simulink model "PI_Controller"  (R2018a)
settings: Solver=VariableStepAuto  StartTime=0.0  StopTime=35  RelTol=1e-3
undefined symbols (not defined in the file): D1, lagging, pulse
libraries: powerlib x12, powerlib_meascontrol x2, simulink x1
settings Model: Creator=Gulten  LastModifiedBy=Gulten

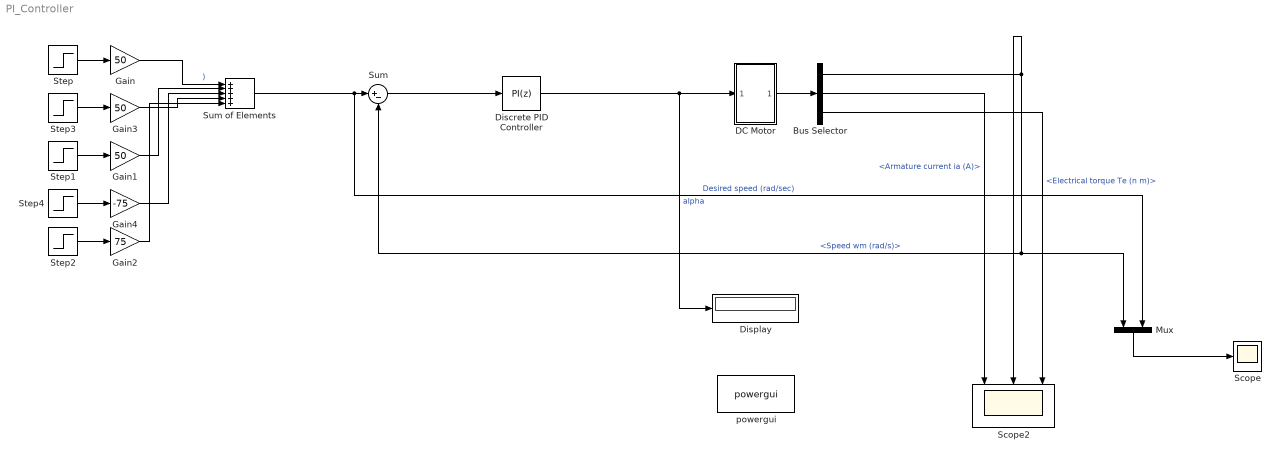
== system PI_Controller ==
  Bus Selector : BusSelector  OutputSignals=Speed wm (rad/s),Armature current ia (A),Electrical torque Te (n m)
  DC Motor : Subsystem
  Discrete PID Controller : simulink/Continuous/PID Controller  Controller=PI  TimeDomain=Discrete-time  SampleTime=0.001  IntegratorMethod=Forward Euler  FilterMethod=Forward Euler  Form=Parallel  UseFilter=on  ControllerParametersSource=internal  P=-2.0474  I=-3.7917  D=0  N=100  InitialConditionSource=internal  InitialConditionForIntegrator=0  InitialConditionForFilter=0  ExternalReset=none  IgnoreLimit=on  LimitOutput=on  UpperSaturationLimit=90  LowerSaturationLimit=0  LinearizeAsGain=off  AntiWindupMode=none  Kb=1  TrackingMode=off  Kt=1  PParamMin=[]  PParamMax=[]  IParamMin=[]  IParamMax=[]  DParamMin=[]  DParamMax=[]  NParamMin=[]  NParamMax=[]  KbParamMin=[]  KbParamMax=[]  KtParamMin=[]  KtParamMax=[]  POutMin=[]  POutMax=[]  IOutMin=[]  IOutMax=[]  DOutMin=[]  DOutMax=[]  NOutMin=[]  NOutMax=[]  KbOutMin=[]  KbOutMax=[]  KtOutMin=[]  KtOutMax=[]  IntegratorOutMin=[]  IntegratorOutMax=[]  FilterOutMin=[]  FilterOutMax=[]  SumOutMin=[]  SumOutMax=[]  SumI1OutMin=[]  SumI1OutMax=[]  SumI2OutMin=[]  SumI2OutMax=[]  SumI3OutMin=[]  SumI3OutMax=[]  SumDOutMin=[]  SumDOutMax=[]  SaturationOutMin=[]  SaturationOutMax=[]  IntegratorContinuousStateAttributes=''  IntegratorStateMustResolveToSignalObject=off  IntegratorRTWStateStorageClass=Auto  FilterContinuousStateAttributes=''  FilterStateMustResolveToSignalObject=off  FilterRTWStateStorageClass=Auto  DifferentiatorICPrevScaledInput=0  DifferentiatorOutMin=[]  DifferentiatorOutMax=[]  FilterDiffOutCoefMin=[]  FilterDiffOutCoefMax=[]  SumDenOutMin=[]  SumDenOutMax=[]  SumNumOutMin=[]  SumNumOutMax=[]  ReciprocalOutMin=[]  ReciprocalOutMax=[]  DivideOutMin=[]  DivideOutMax=[]  TunerSelectOption=Frequency Response Based
  Display : Display
  Gain : Gain  Gain=50
  Gain1 : Gain  Gain=50
  Gain2 : Gain  Gain=75
  Gain3 : Gain  Gain=50
  Gain4 : Gain  Gain=-75
  Mux : Mux  Inputs=2
  Scope : Scope
  Scope2 : Scope  NumInputPorts=3
  Step : Step  Time=0  SampleTime=0
  Step1 : Step  Time=5  SampleTime=0
  Step2 : Step  Time=25  SampleTime=0
  Step3 : Step  Time=3  SampleTime=0
  Step4 : Step  Time=15  SampleTime=0
  Sum : Sum  Inputs=|+-
  Sum of Elements : Sum  Inputs=+++++
  powergui : powerlib/powergui  Priority=1  SimulationMode=Discrete  SampleTime=10e-6  frequency=60  Iterations=50  frequencyindice=50  Pbase=100e6  ErrMax=1e-4  UnitsV=kV  UnitsW=MW  buscounter=0  FunctionMessages=off  echomessages=off  EnableUseOfTLC=off  CurrentSourceSwitches=off  DisableSnubberDevices=off  DisableRonSwitches=off  DisableVfSwitches=off  DisplayEquations=off  SolverType=Tustin/Backward Euler (TBE)  Interpol=off  ExternalGateDelay=off  methode=off  Ts=100  x0status=blocks  SPID=on  SwTol=0  HookPort=off  RestoreLinks=warning  ResistiveCurrentMeasurement=off  Frange=[0:2:500]  Ylog=off  Xlog=on  ShowGrid=off  save=off  variable=ZData  structure=ScopeData  ZoomFFT=on  StartTime=3  cycles=10  DisplayStyle=1  fundamental=50  FreqAxis=on  MaxFrequency=1000  frequencyindicesteady=1  RmsSteady=1  display=off
  wires:
  Bus Selector/3 -> Scope2/3  "<Electrical torque Te (n m)>"
  Bus Selector/1 -> Scope2/2, Mux/1, Sum/2  "<Speed wm (rad/s)>"
  Bus Selector/2 -> Scope2/1  "<Armature current ia (A)>"
  DC Motor/1(Out1) -> Bus Selector/1
  Step/1 -> Gain/1
  Mux/1 -> Scope/1
  Step1/1 -> Gain1/1
  Step2/1 -> Gain2/1
  Gain/1 -> Sum of Elements/1  ")"
  Gain1/1 -> Sum of Elements/2
  Gain2/1 -> Sum of Elements/5
  Sum of Elements/1 -> Mux/2, Sum/1  "Desired speed (rad/sec)"
  Discrete PID Controller/1 -> Display/1, DC Motor/1(In1)  "alpha"
  Sum/1 -> Discrete PID Controller/1
  Step3/1 -> Gain3/1
  Gain3/1 -> Sum of Elements/4
  Step4/1 -> Gain4/1
  Gain4/1 -> Sum of Elements/3

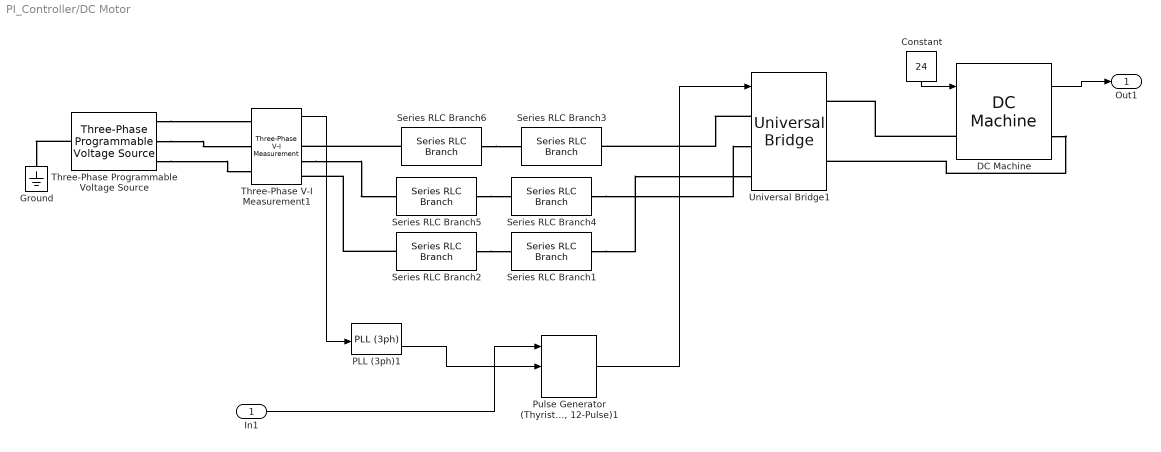
== system PI_Controller/DC Motor ==
  In1 : Inport
  Constant : Constant  Value=24
  DC Machine : powerlib/Machines/DC Machine  PresetModel=No  MechanicalLoad=Torque TL  FieldType=Permanent magnet  ShowDetailedParameters=on  MeasurementBus=off  RLa=[ 10 0.01]  RLf="[ 240  120]"  Laf=1.8  MachineConstant=Back-emf constant (V/rpm)  Ke=0.3  Kt=1.8  J=0.4  Bm=0  Tf=0  w0=1  Ifinit=1  TsPowergui=0  TsBlock=-1
  Ground : powerlib/Elements/Ground  LConnTagsString=a
  PLL (3ph)1 : powerlib_meascontrol/PLL/PLL (3ph)  Fmin=45  Par_Init=[0, 60]  ParK=[180, 3200, 1]  TcD=1e-4  MaxRateChangeFreq=12  FilterCutOffFreq=25  Ts=0  AGC=on
  "Pulse Generator (Thyristor, 12-Pulse)1" : powerlib_meascontrol/Pulse & Signal Generators/Pulse Generator (Thyristor, 12-Pulse)  GenType=6-pulse  Delta=D1 (lagging)  pwidth=60  Double_Pulse=off  Ts=1e-5
      settings: SourceProductName=Simscape Power Systems  SourceProductBaseCode=PS
  Series RLC Branch1 : powerlib/Elements/Series RLC Branch  LConnTagsString=__new0  RConnTagsString=__new0  BranchType=L  Resistance=1  Inductance=100e-6  SetiL0=off  InitialCurrent=0  Capacitance=1e-6  Setx0=off  InitialVoltage=0  Measurements=None
  Series RLC Branch2 : powerlib/Elements/Series RLC Branch  LConnTagsString=__new0  RConnTagsString=__new0  BranchType=R  Resistance=0.1  Inductance=1e-3  SetiL0=off  InitialCurrent=0  Capacitance=1e-6  Setx0=off  InitialVoltage=0  Measurements=None
  Series RLC Branch3 : powerlib/Elements/Series RLC Branch  LConnTagsString=__new0  RConnTagsString=__new0  BranchType=L  Resistance=1  Inductance=100e-6  SetiL0=off  InitialCurrent=0  Capacitance=1e-6  Setx0=off  InitialVoltage=0  Measurements=None
  Series RLC Branch4 : powerlib/Elements/Series RLC Branch  LConnTagsString=__new0  RConnTagsString=__new0  BranchType=L  Resistance=1  Inductance=100e-6  SetiL0=off  InitialCurrent=0  Capacitance=1e-6  Setx0=off  InitialVoltage=0  Measurements=None
  Series RLC Branch5 : powerlib/Elements/Series RLC Branch  LConnTagsString=__new0  RConnTagsString=__new0  BranchType=R  Resistance=0.1  Inductance=1e-3  SetiL0=off  InitialCurrent=0  Capacitance=1e-6  Setx0=off  InitialVoltage=0  Measurements=None
  Series RLC Branch6 : powerlib/Elements/Series RLC Branch  LConnTagsString=__new0  RConnTagsString=__new0  BranchType=R  Resistance=0.1  Inductance=1e-3  SetiL0=off  InitialCurrent=0  Capacitance=1e-6  Setx0=off  InitialVoltage=0  Measurements=None
  Three-Phase Programmable Voltage Source : powerlib/Electrical Sources/Three-Phase Programmable Voltage Source  PositiveSequence="[400  0 50]"  VariationEntity=None  VariationType=Table of time-amplitude pairs  VariationTypeAlt=Step  VariationStep=0.5  VariationRate=10  VariationMagnitude=0.3  VariationFrequency=2  VariationTiming=[1 2]  VariationPhaseA=off  Amplitudes=[1 0.8 1.2 1.0]  TimeValues=[0 0.1 0.15 0.2]  HarmonicGeneration=off  HarmonicA=[3 0.2 -25 0]  HarmonicB=[2 0.15 35 2]  Timing="[0.05  3]"  BusType=swing  Pref=0  Qref=0  Qmin=-inf  Qmax=inf
  Three-Phase V-I Measurement1 : powerlib/Measurements/Three-Phase V-I Measurement  VoltageMeasurement=phase-to-ground  SetLabelV=off  LabelV=Vabc  Vpu=off  VpuLL=off  CurrentMeasurement=yes  SetLabelI=off  LabelI=Iabc  Ipu=off  Pbase=100e6  Vbase=500e3  OutputType=Complex  PhasorSimulation=off  PSBequivalent=0
  Universal Bridge1 : powerlib/Power Electronics/Universal Bridge  Arms=3  SnubberResistance=1e5  SnubberCapacitance=inf  Device=Thyristors  Ron=0.020  Lon=0  ForwardVoltages="[  0  0  ]"  ForwardVoltage=0.8  GTOparameters=[ 10e-6 , 20e-6 ]  IGBTparameters=[ 1e-6 , 2e-6 ]  Measurements=None  Measurements_2=None  converterType=Rectifier
  Out1 : Outport
  wires:
  Constant/1 -> DC Machine/1
  "Pulse Generator (Thyristor, 12-Pulse)1"/1 -> Universal Bridge1/1
  PLL (3ph)1/2 -> "Pulse Generator (Thyristor, 12-Pulse)1"/2
  Three-Phase V-I Measurement1/1 -> PLL (3ph)1/1
  DC Machine/1 -> Out1/1
  In1/1 -> "Pulse Generator (Thyristor, 12-Pulse)1"/1
  connections:
  DC Machine/RConn1 -- Universal Bridge1/RConn2
  Series RLC Branch1/LConn1 -- Universal Bridge1/LConn3
  Three-Phase Programmable Voltage Source/RConn2 -- Three-Phase V-I Measurement1/LConn2
  Series RLC Branch6/LConn1 -- Series RLC Branch3/RConn1
  Universal Bridge1/LConn1 -- Series RLC Branch3/LConn1
  Series RLC Branch5/LConn1 -- Series RLC Branch4/RConn1
  Three-Phase Programmable Voltage Source/LConn1 -- Ground/LConn1
  Series RLC Branch2/RConn1 -- Three-Phase V-I Measurement1/RConn3
  DC Machine/LConn1 -- Universal Bridge1/RConn1
  Series RLC Branch6/RConn1 -- Three-Phase V-I Measurement1/RConn1
  Three-Phase V-I Measurement1/RConn2 -- Series RLC Branch5/RConn1
  Series RLC Branch2/LConn1 -- Series RLC Branch1/RConn1
  Three-Phase Programmable Voltage Source/RConn1 -- Three-Phase V-I Measurement1/LConn1
  Series RLC Branch4/LConn1 -- Universal Bridge1/LConn2
  Three-Phase Programmable Voltage Source/RConn3 -- Three-Phase V-I Measurement1/LConn3
